simulink model "Control_PWM_Pulmon"  (R2018a)
settings: Solver=VariableStepAuto  StartTime=0.0  StopTime=10.0  RelTol=1e-3
libraries: simulink x3, pePwmGenerator x1
settings Model: Creator=Ruben  LastModifiedBy=Ruben

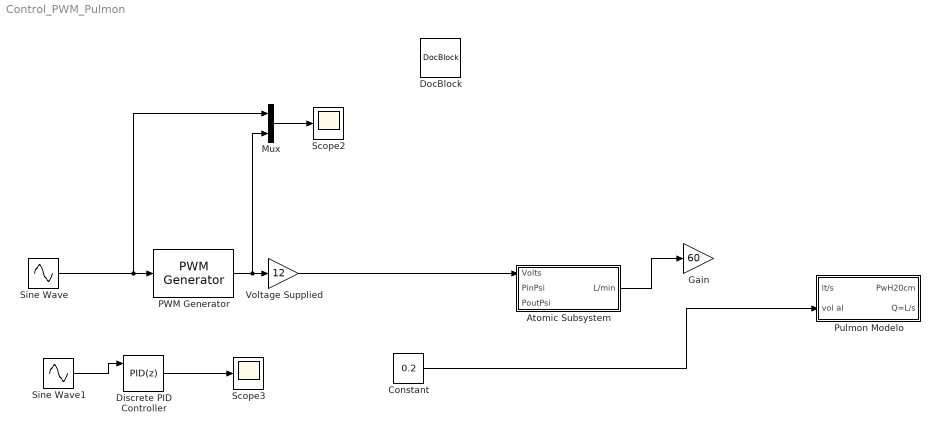
== system Control_PWM_Pulmon ==
  Atomic Subsystem : Subsystem  TreatAsAtomicUnit=on
  Constant : Constant  Value=0.2
  Discrete PID Controller : simulink/Continuous/PID Controller  Controller=PID  TimeDomain=Discrete-time  SampleTime=.1  IntegratorMethod=Forward Euler  FilterMethod=Forward Euler  Form=Parallel  UseFilter=on  ControllerParametersSource=internal  P=1  I=1  D=0  N=100  InitialConditionSource=internal  InitialConditionForIntegrator=0  InitialConditionForFilter=0  ExternalReset=rising  LimitOutput=off  UpperSaturationLimit=inf  LowerSaturationLimit=-inf  LinearizeAsGain=off  AntiWindupMode=none  Kb=1  TrackingMode=off  Kt=1  PParamMin=[]  PParamMax=[]  IParamMin=[]  IParamMax=[]  DParamMin=[]  DParamMax=[]  NParamMin=[]  NParamMax=[]  KbParamMin=[]  KbParamMax=[]  KtParamMin=[]  KtParamMax=[]  POutMin=[]  POutMax=[]  IOutMin=[]  IOutMax=[]  DOutMin=[]  DOutMax=[]  NOutMin=[]  NOutMax=[]  KbOutMin=[]  KbOutMax=[]  KtOutMin=[]  KtOutMax=[]  IntegratorOutMin=[]  IntegratorOutMax=[]  FilterOutMin=[]  FilterOutMax=[]  SumOutMin=[]  SumOutMax=[]  SumI1OutMin=[]  SumI1OutMax=[]  SumI2OutMin=[]  SumI2OutMax=[]  SumI3OutMin=[]  SumI3OutMax=[]  SumDOutMin=[]  SumDOutMax=[]  SaturationOutMin=[]  SaturationOutMax=[]  IntegratorContinuousStateAttributes=''  IntegratorStateMustResolveToSignalObject=off  IntegratorRTWStateStorageClass=Auto  FilterContinuousStateAttributes=''  FilterStateMustResolveToSignalObject=off  FilterRTWStateStorageClass=Auto  DifferentiatorICPrevScaledInput=0  DifferentiatorOutMin=[]  DifferentiatorOutMax=[]  FilterDiffOutCoefMin=[]  FilterDiffOutCoefMax=[]  SumDenOutMin=[]  SumDenOutMax=[]  SumNumOutMin=[]  SumNumOutMax=[]  ReciprocalOutMin=[]  ReciprocalOutMax=[]  DivideOutMin=[]  DivideOutMax=[]  TunerSelectOption=Transfer Function Based (PID Tuner App)
  DocBlock : simulink/Model-Wide Utilities/DocBlock  DocumentType=Text
      content=|
      | %mechanical partvalve modeling as Flux=k*i*delta P(static_Gain/(Ts+1))
      | %k=
  Gain : Gain  Gain=60
  Mux : Mux  Inputs=2
  PWM Generator : pePwmGenerator/PWM Generator  CarrCount=Up  Tper=0.1  Ts=5e-5
  Pulmon Modelo : Subsystem  TreatAsAtomicUnit=on
  Scope2 : Scope
  Scope3 : Scope
  Sine Wave : Sin  Amplitude=.5  Bias=.5  Frequency=30  SampleTime=0
  Sine Wave1 : Sin  Amplitude=.5  Bias=.5  Frequency=30  SampleTime=0
  Voltage Supplied : Gain  Gain=12
  wires:
  Sine Wave/1 -> Mux/1, PWM Generator/1
  PWM Generator/1 -> Mux/2, Voltage Supplied/1
  Voltage Supplied/1 -> Atomic Subsystem/1("Volts ")
  Mux/1 -> Scope2/1
  Sine Wave1/1 -> Discrete PID Controller/1
  Discrete PID Controller/1 -> Scope3/1
  Constant/1 -> Pulmon Modelo/2(vol al)
  Atomic Subsystem/1(L/min) -> Gain/1

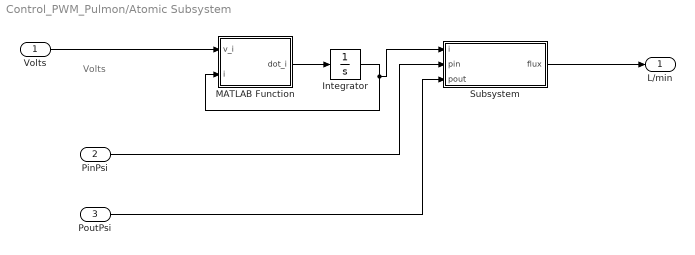
== system Control_PWM_Pulmon/Atomic Subsystem ==
  note: Volts
  "Volts " : Inport
  PinPsi : Inport  Port=2
  PoutPsi : Inport  Port=3
  Integrator : Integrator
  MATLAB Function : MATLAB Function  TreatAsAtomicUnit=on
  Subsystem : Subsystem
  L/min : Outport
  wires:
  Integrator/1 -> Subsystem/1(i), MATLAB Function/2(i)
  MATLAB Function/1(dot_i) -> Integrator/1
  "Volts "/1 -> MATLAB Function/1(v_i)
  Subsystem/1(flux) -> L/min/1
  PinPsi/1 -> Subsystem/2(pin)
  PoutPsi/1 -> Subsystem/3(pout)

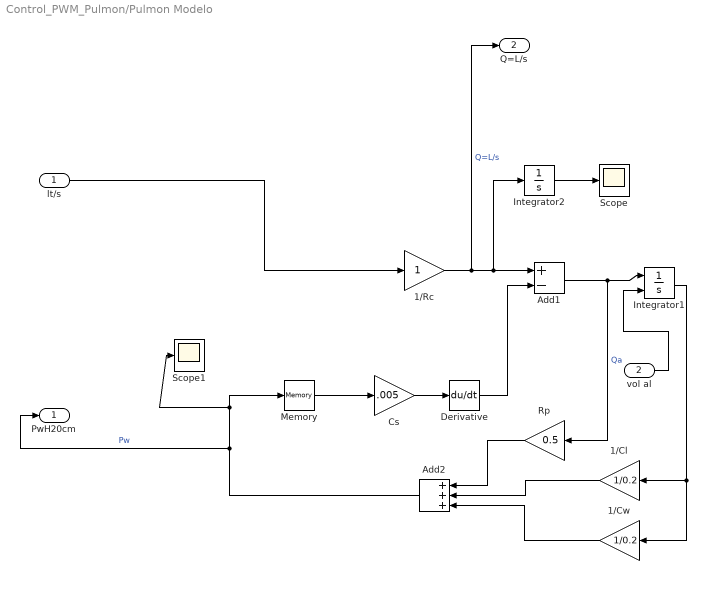
== system Control_PWM_Pulmon/Pulmon Modelo ==
  lt/s : Inport
  vol al : Inport  Port=2
  1/Cl : Gain  Gain=1/0.2
  1/Cw : Gain  Gain=1/0.2
  1/Rc : Gain
  Add1 : Sum  Inputs=+-
  Add2 : Sum  Inputs=+++
  Cs : Gain  Gain=.005
  Derivative : Derivative
  Integrator1 : Integrator  InitialConditionSource=external  ContinuousStateAttributes=volumen
  Integrator2 : Integrator
  Memory : Memory
  Rp : Gain  Gain=0.5
  Scope : Scope
  Scope1 : Scope
  PwH20cm : Outport
  Q=L/s : Outport  Port=2
  wires:
  Add1/1 -> Rp/1, Integrator1/1  "Qa"
  Derivative/1 -> Add1/2
  1/Rc/1 -> Q=L/s/1, Integrator2/1, Add1/1  "Q=L/s"
  Cs/1 -> Derivative/1
  Memory/1 -> Cs/1
  1/Cw/1 -> Add2/3
  Integrator2/1 -> Scope/1
  Rp/1 -> Add2/1
  1/Cl/1 -> Add2/2
  Add2/1 -> Scope1/1, Memory/1, PwH20cm/1  "Pw"
  Integrator1/1 -> 1/Cw/1, 1/Cl/1
  lt/s/1 -> 1/Rc/1
  vol al/1 -> Integrator1/2

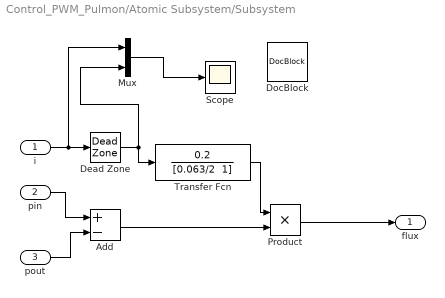
== system Control_PWM_Pulmon/Atomic Subsystem/Subsystem ==
  i : Inport
  pin : Inport  Port=2
  pout : Inport  Port=3
  Add : Sum  Inputs=+-
  Dead Zone : DeadZone  LowerValue=0  UpperValue=.250  SaturateOnIntegerOverflow=on
  DocBlock : simulink/Model-Wide Utilities/DocBlock  DocumentType=Text
      content=|
      | flux=k*I*deltaP
      |  delay = 1/(Ts+1)
      |
      | k=delta flux/ delta i % de tablas aprox 20/100
      | T=L/R  L=0.063
      | R=2
      | dead zone =250 promedio
      | %flux slpm
      | Delta P en PSI
  Mux : Mux  Inputs=2
  Product : Product
  Scope : Scope
  Transfer Fcn : TransferFcn  Numerator=[0.2]  Denominator="[0.063/2  1]"
  flux : Outport
  wires:
  pin/1 -> Add/1
  pout/1 -> Add/2
  Add/1 -> Product/2
  Transfer Fcn/1 -> Product/1
  Product/1 -> flux/1
  i/1 -> Mux/1, Dead Zone/1
  Dead Zone/1 -> Transfer Fcn/1, Mux/2
  Mux/1 -> Scope/1

== matlab function Control_PWM_Pulmon/Atomic Subsystem/MATLAB Function ==
  data: v_i input; dot_i output; i input
function dot_i = fcn(v_i,i)
R=20; % R igual a 2 ohm
L=.063 ;% L aprox 63mh
dot_i = (1/L)*(v_i-R*i);
